simulink model "trans_line_2"  (Simulink 7.4)
settings: Solver=ode45  StartTime=0.0  StopTime=1e-7  MaxStep=.05e-9;  RelTol=1e-3
libraries: powerlib x10, simulink x1
settings Model: Creator=dbenson  LastModifiedBy=Dick
settings OptimizationCC: InitFltsAndDblsToZero=on
settings DebuggingCC: SaveWithParameterizedLinksMsg=none  SignalResolutionControl=TryResolveAllWithWarning  MultiTaskDSMMsg=warning  MultiTaskCondExecSysMsg=none
settings RTWCC: IncludeERTFirstTime=on
settings GRTTargetCC: TargetFcnLib=ansi_tfl_tmw.mat

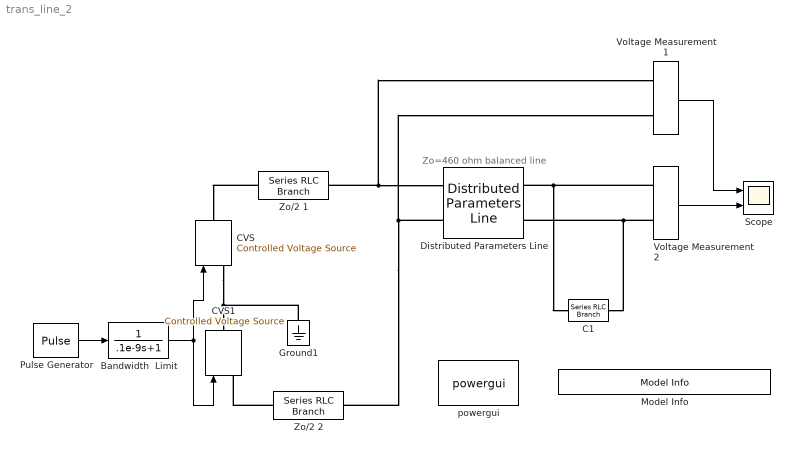
== system trans_line_2 ==
  note: Zo=460 ohm balanced line
  Bandwidth  Limit : TransferFcn  Denominator=[.1e-9 1]
  C1 : powerlib/Elements/Series RLC Branch  DialogController=POWERSYS.PowerSysDialog  PhysicalDomain=powersysdomain  SubClassName=unknown  LeftPortType=p1  RightPortType=p1  LConnTagsString=__new0  RConnTagsString=__new0  BranchType=C  Resistance=1  Inductance=1e-3  SetiL0=off  InitialCurrent=0  Capacitance=0.1e-12  Setx0=off  InitialVoltage=0  Measurements=None
  CVS : powerlib/Electrical Sources/Controlled Voltage Source  DialogController=POWERSYS.PowerSysDialog  SystemSampleTime=-1  Initialize=on  Source_Type=DC  Amplitude=0  Phase=0  Frequency=0  Measurements=None
  CVS1 : powerlib/Electrical Sources/Controlled Voltage Source  DialogController=POWERSYS.PowerSysDialog  SystemSampleTime=-1  Initialize=on  Source_Type=DC  Amplitude=0  Phase=0  Frequency=0  Measurements=None
  Distributed Parameters Line : powerlib/Elements/Distributed Parameters Line  DialogController=POWERSYS.PowerSysDialog  SystemSampleTime=-1  Phases=2  Frequency=1000000  Resistance=[33.362 30.175;30.175 33.362]  Inductance=[0.0010569 0.00028823;0.00028823 0.0010569]  Capacitance=[1.141e-008 -3.0743e-009;-3.0743e-009 1.141e-008]  Length=.001  x1=[0 0 0;6.6970441661975e-010 0 0;1.3394088332395e-009 0 0;2.00911324985925e-009 0 0;2.678817666479e-009 0 0;3.34852208309875e-009 0 0]  x2=[0 0 0;6.6970441661975e-010 0 0;1.3394088332395e-009 0 0;2.00911324985925e-009 0 0;2.678817666479e-009 0 0;3.34852208309875e-009 0 0]  x3=[0 0 0;6.6970441661975e-010 0 0;1.3394088332395e-009 0 0;2.00911324985925e-009 0 0;2.678817666479e-009 0 0;3.34852208309875e-009 0 0]  x4=[0 0 0;6.6970441661975e-010 0 0;1.3394088332395e-009 0 0;2.00911324985925e-009 0 0;2.678817666479e-009 0 0;3.34852208309875e-009 0 0]  x5=3.34852208309875e-009  Measurements=None
  Ground1 : powerlib/Elements/Ground  DialogController=POWERSYS.PowerSysDialog  PhysicalDomain=powersysdomain  SubClassName=unknown  LeftPortType=p1  RightPortType=p1  LConnTagsString=a
  Model Info : simulink/Model-Wide Utilities/Model Info  SystemSampleTime=-1  InitialBlockCM=None  BlockCM=None  Frame=on  DisplayStringWithTags=Copywrite 2005-2010 The MathWorks, Inc.  HorizontalTextAlignment=Center  LeftAlignmentValue=0.5  SourceBlockDiagram=trans_line_2  TagMaxNumber=20
  Pulse Generator : DiscretePulseGenerator  PulseType=Time based  Amplitude=1  Period=0.5e-7  PulseWidth=50  PhaseDelay=0  SampleTime=1
  Scope : Scope  NumInputPorts=2
      settings: YMin=-5~-5  YMax=5~5
  Voltage Measurement1 : powerlib/Measurements/Voltage Measurement  DialogController=POWERSYS.PowerSysDialog  SystemSampleTime=-1  PhasorSimulation=off  OutputType=Complex  PSBequivalent=0
  Voltage Measurement2 : powerlib/Measurements/Voltage Measurement  DialogController=POWERSYS.PowerSysDialog  SystemSampleTime=-1  PhasorSimulation=off  OutputType=Complex  PSBequivalent=0
  Zo/2 1 : powerlib/Elements/Series RLC Branch  DialogController=POWERSYS.PowerSysDialog  PhysicalDomain=powersysdomain  SubClassName=unknown  LeftPortType=p1  RightPortType=p1  LConnTagsString=__new0  RConnTagsString=__new0  BranchType=R  Resistance=460.7/2  Inductance=1e-3  SetiL0=off  InitialCurrent=0  Capacitance=1e-6  Setx0=off  InitialVoltage=0  Measurements=None
  Zo/2 2 : powerlib/Elements/Series RLC Branch  DialogController=POWERSYS.PowerSysDialog  PhysicalDomain=powersysdomain  SubClassName=unknown  LeftPortType=p1  RightPortType=p1  LConnTagsString=__new0  RConnTagsString=__new0  BranchType=R  Resistance=460.7/2  Inductance=1e-3  SetiL0=off  InitialCurrent=0  Capacitance=1e-6  Setx0=off  InitialVoltage=0  Measurements=None
  powergui : powerlib/powergui  SystemSampleTime=-1  SimulationMode=Continuous  SampleTime=50e-6  frequency=60  SPID=off  DisableSnubberDevices=off  DisableRonSwitches=off  DisableVfSwitches=off  SwTol=0  Interpol=off  frequencyindice=0  echomessages=off  HookPort=off  DisplayEquations=off  FunctionMessages=off  EnableUseOfTLC=off  x0status=blocks  RestoreLinks=warning  Frange=[0:2:500]  Ylog=off  Xlog=on  ShowGrid=off  save=off  variable=ZData  ZoomFFT=on  StartTime=0.0  cycles=1  DisplayStyle=1  fundamental=60  FreqAxis=off  MaxFrequency=1000  frequencyindicesteady=1  RmsSteady=1  display=off  Ts=0  methode=off
  wires:
  Pulse Generator/1 -> Bandwidth  Limit/1
  Bandwidth  Limit/1 -> CVS/1, CVS1/1
  Voltage Measurement2/1 -> Scope/2
  Voltage Measurement1/1 -> Scope/1
  connections:
  Zo/2 1/RConn1 -- Distributed Parameters Line/LConn1 -- Voltage Measurement1/LConn1
  Zo/2 1/LConn1 -- CVS/RConn1
  Voltage Measurement2/LConn1 -- Distributed Parameters Line/RConn1 -- C1/LConn1
  Voltage Measurement2/LConn2 -- Distributed Parameters Line/RConn2 -- C1/RConn1
  Zo/2 2/LConn1 -- CVS1/LConn1
  Zo/2 2/RConn1 -- Distributed Parameters Line/LConn2 -- Voltage Measurement1/LConn2
  Ground1/LConn1 -- CVS/LConn1 -- CVS1/RConn1
